simulink model "Zad2manipulator"  (R2025a)
settings: Solver=VariableStepAuto  StartTime=0.0  StopTime=10  RelTol=1e-3
values from neighbouring files (symbols this model uses):
  B1 = 2    [Zad2_manipulator.m]
  B2 = 2    [Zad2_manipulator.m]
  final_uhol = -pi/4    (= -0.785398163397)    [Zad2_manipulator.m]
  g = 9.81    [Zad2_manipulator.m]
  l1 = 0.25    [Zad2_manipulator.m]
  l2 = 0.25    [Zad2_manipulator.m]
  m1 = 3    [Zad2_manipulator.m]
  m2 = 3    [Zad2_manipulator.m]
libraries: slpidlib x2
settings Model: Creator=MATÚŠ  LastModifiedBy=MATÚŠ

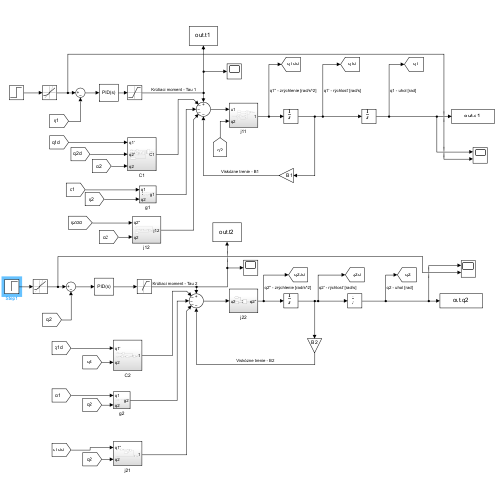
[thumbnail: Simulink's stored preview of the top-level diagram]
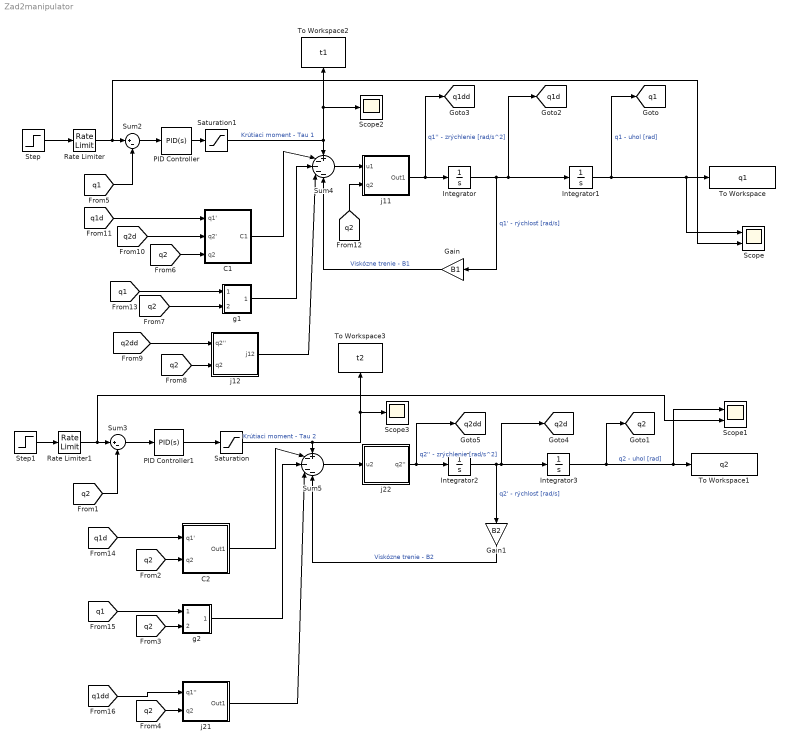
== system Zad2manipulator ==
  C1 : Subsystem
  C2 : Subsystem
  Gain : Gain  Gain=B1
  Gain1 : Gain  Gain=B2
  Integrator : Integrator
  Integrator1 : Integrator  InitialCondition=-pi/2
  Integrator2 : Integrator
  Integrator3 : Integrator  InitialCondition=-pi/2
  PID Controller : slpidlib/PID Controller  Controller=PID  Form=Parallel  TimeDomain=Continuous-time  UseExternalTs=off  SampleTime=-1  IntegratorMethod=Forward Euler  FilterMethod=Forward Euler  ControllerParametersSource=internal  P=300  I=300  UseKiTs=off  D=30  UseExternalDerivativeSource=off  N=300  UseFilter=on  TunerSelectOption=Transfer Function Based (PID Tuner App)  InitialConditionSource=internal  InitialConditionForIntegrator=0  InitialConditionForFilter=0  DifferentiatorICPrevScaledInput=0  ExternalReset=none  TrackingMode=off  Kt=1  LimitOutput=off  SatLimitsSource=internal  UpperSaturationLimit=inf  LowerSaturationLimit=-inf  LinearizeAsGain=on  AntiWindupMode=none  Kb=1  LimitIntegrator=off  UpperIntegratorSaturationLimit=inf  LowerIntegratorSaturationLimit=-inf  POutMin=[]  POutMax=[]  IOutMin=[]  IOutMax=[]  DOutMin=[]  DOutMax=[]  NOutMin=[]  NOutMax=[]  SumOutMin=[]  SumOutMax=[]  SaturationOutMin=[]  SaturationOutMax=[]  PParamMin=[]  PParamMax=[]  IParamMin=[]  IParamMax=[]  DParamMin=[]  DParamMax=[]  NParamMin=[]  NParamMax=[]  KbParamMin=[]  KbParamMax=[]  KtParamMin=[]  KtParamMax=[]  KbOutMin=[]  KbOutMax=[]  KtOutMin=[]  KtOutMax=[]  IntegratorOutMin=[]  IntegratorOutMax=[]  FilterOutMin=[]  FilterOutMax=[]  SumI1OutMin=[]  SumI1OutMax=[]  SumI2OutMin=[]  SumI2OutMax=[]  SumI3OutMin=[]  SumI3OutMax=[]  SumI4OutMin=[]  SumI4OutMax=[]  SumDOutMin=[]  SumDOutMax=[]  DifferentiatorOutMin=[]  DifferentiatorOutMax=[]  FilterDiffOutCoefMin=[]  FilterDiffOutCoefMax=[]  ReciprocalOutMin=[]  ReciprocalOutMax=[]  SumDenOutMin=[]  SumDenOutMax=[]  SumNumOutMin=[]  SumNumOutMax=[]  DivideOutMin=[]  DivideOutMax=[]  UdiffTsProdOutMin=[]  UdiffTsProdOutMax=[]  NTsProdOutMin=[]  NTsProdOutMax=[]  UintegralTsProdOutMin=[]  UintegralTsProdOutMax=[]  UngainTsProdOutMin=[]  UngainTsProdOutMax=[]  ClampingZeroOutDataTypeStr=Inherit: Inherit via back propagation  ClampingZeroOutMin=[]  ClampingZeroOutMax=[]  FilterDenConstantOutDataTypeStr=Inherit: Inherit via back propagation  FilterDenConstantOutMin=[]  FilterDenConstantOutMax=[]  PCopyOutDataTypeStr=Inherit: Inherit via back propagation  PCopyOutMin=[]  PCopyOutMax=[]  NCopyOutDataTypeStr=Inherit: Inherit via back propagation  NCopyOutMin=[]  NCopyOutMax=[]  IntegratorContinuousStateAttributes=''  IntegratorStateMustResolveToSignalObject=off  IntegratorRTWStateStorageClass=Auto  FilterContinuousStateAttributes=''  FilterStateMustResolveToSignalObject=off  FilterRTWStateStorageClass=Auto  ParallelPVariant=InternalParameters  IdealPVariant=Disabled  IVariant=InternalParameters  DVariant=InternalParameters  IntegratorVariant=Continuous  SatVariant=Disabled  AWVariant=Passthrough  PCopyVariant=Disabled  TRVariant=Disabled  FdbkBlocksVariant=Forward  IdealPFdbkVariant=Disabled  SatFdbkVariant=Disabled  DerivativeFilterVariant=ContFilter  NVariant=InternalParameters  NCopyVariant=Disabled  FilterICVariant=InternalICsFilter  IntegratorICVariant=InternalICs  ExternalResetVariant=Disabled  TRSumVariant=Passthrough  SumFdbkVariant=Disabled  SumVariant=Sum_PID  TsampFilterVariant=InternalTs  TsampNgainVariant=Passthrough  TsampIntegralVariant=Disabled_SignalSpec  ExternalSaturationOutDataTypeStr=Inherit: Same as second input  DerivativeSourceVariant=ErrorSignal  PreIntVariant=InternalPreInt
  PID Controller1 : slpidlib/PID Controller  Controller=PID  Form=Parallel  TimeDomain=Continuous-time  UseExternalTs=off  SampleTime=-1  IntegratorMethod=Forward Euler  FilterMethod=Forward Euler  ControllerParametersSource=internal  P=300  I=300  UseKiTs=off  D=30  UseExternalDerivativeSource=off  N=300  UseFilter=on  TunerSelectOption=Transfer Function Based (PID Tuner App)  InitialConditionSource=internal  InitialConditionForIntegrator=0  InitialConditionForFilter=0  DifferentiatorICPrevScaledInput=0  ExternalReset=none  TrackingMode=off  Kt=1  LimitOutput=off  SatLimitsSource=internal  UpperSaturationLimit=inf  LowerSaturationLimit=-inf  LinearizeAsGain=on  AntiWindupMode=none  Kb=1  LimitIntegrator=off  UpperIntegratorSaturationLimit=inf  LowerIntegratorSaturationLimit=-inf  POutMin=[]  POutMax=[]  IOutMin=[]  IOutMax=[]  DOutMin=[]  DOutMax=[]  NOutMin=[]  NOutMax=[]  SumOutMin=[]  SumOutMax=[]  SaturationOutMin=[]  SaturationOutMax=[]  PParamMin=[]  PParamMax=[]  IParamMin=[]  IParamMax=[]  DParamMin=[]  DParamMax=[]  NParamMin=[]  NParamMax=[]  KbParamMin=[]  KbParamMax=[]  KtParamMin=[]  KtParamMax=[]  KbOutMin=[]  KbOutMax=[]  KtOutMin=[]  KtOutMax=[]  IntegratorOutMin=[]  IntegratorOutMax=[]  FilterOutMin=[]  FilterOutMax=[]  SumI1OutMin=[]  SumI1OutMax=[]  SumI2OutMin=[]  SumI2OutMax=[]  SumI3OutMin=[]  SumI3OutMax=[]  SumI4OutMin=[]  SumI4OutMax=[]  SumDOutMin=[]  SumDOutMax=[]  DifferentiatorOutMin=[]  DifferentiatorOutMax=[]  FilterDiffOutCoefMin=[]  FilterDiffOutCoefMax=[]  ReciprocalOutMin=[]  ReciprocalOutMax=[]  SumDenOutMin=[]  SumDenOutMax=[]  SumNumOutMin=[]  SumNumOutMax=[]  DivideOutMin=[]  DivideOutMax=[]  UdiffTsProdOutMin=[]  UdiffTsProdOutMax=[]  NTsProdOutMin=[]  NTsProdOutMax=[]  UintegralTsProdOutMin=[]  UintegralTsProdOutMax=[]  UngainTsProdOutMin=[]  UngainTsProdOutMax=[]  ClampingZeroOutDataTypeStr=Inherit: Inherit via back propagation  ClampingZeroOutMin=[]  ClampingZeroOutMax=[]  FilterDenConstantOutDataTypeStr=Inherit: Inherit via back propagation  FilterDenConstantOutMin=[]  FilterDenConstantOutMax=[]  PCopyOutDataTypeStr=Inherit: Inherit via back propagation  PCopyOutMin=[]  PCopyOutMax=[]  NCopyOutDataTypeStr=Inherit: Inherit via back propagation  NCopyOutMin=[]  NCopyOutMax=[]  IntegratorContinuousStateAttributes=''  IntegratorStateMustResolveToSignalObject=off  IntegratorRTWStateStorageClass=Auto  FilterContinuousStateAttributes=''  FilterStateMustResolveToSignalObject=off  FilterRTWStateStorageClass=Auto  ParallelPVariant=InternalParameters  IdealPVariant=Disabled  IVariant=InternalParameters  DVariant=InternalParameters  IntegratorVariant=Continuous  SatVariant=Disabled  AWVariant=Passthrough  PCopyVariant=Disabled  TRVariant=Disabled  FdbkBlocksVariant=Forward  IdealPFdbkVariant=Disabled  SatFdbkVariant=Disabled  DerivativeFilterVariant=ContFilter  NVariant=InternalParameters  NCopyVariant=Disabled  FilterICVariant=InternalICsFilter  IntegratorICVariant=InternalICs  ExternalResetVariant=Disabled  TRSumVariant=Passthrough  SumFdbkVariant=Disabled  SumVariant=Sum_PID  TsampFilterVariant=InternalTs  TsampNgainVariant=Passthrough  TsampIntegralVariant=Disabled_SignalSpec  ExternalSaturationOutDataTypeStr=Inherit: Same as second input  DerivativeSourceVariant=ErrorSignal  PreIntVariant=InternalPreInt
  Rate Limiter : RateLimiter  SampleTimeMode=inherited
  Rate Limiter1 : RateLimiter  SampleTimeMode=inherited
  Saturation : Saturate  UpperLimit=15  LowerLimit=-15
  Saturation1 : Saturate  UpperLimit=30  LowerLimit=-30
  Scope : Scope  NumInputPorts=2
      settings: ActiveDisplayYMinimum=-1  ActiveDisplayYMaximum=1
  Scope1 : Scope  NumInputPorts=2
      settings: ActiveDisplayYMinimum=-1.2681933125497675  ActiveDisplayYMaximum=0.63598203377017948
  Scope2 : Scope
      settings: ActiveDisplayYMinimum=-1  ActiveDisplayYMaximum=1  DataLoggingVariableName=ScopeData2
  Scope3 : Scope
      settings: DataLoggingVariableName=ScopeData3
  Step : Step  Time=pi/4  Before=-pi/2  After=final_uhol  SampleTime=0
  Step1 : Step  Time=pi/4  Before=-pi/2  After=final_uhol  SampleTime=0
  Sum2 : Sum  Inputs=|+-
  Sum3 : Sum  Inputs=|+-
  Sum4 : Sum  Inputs=+----
  Sum5 : Sum  Inputs=+----
  To Workspace : ToWorkspace  VariableName=q1  SaveFormat=Structure With Time  SampleTime=-1
  To Workspace1 : ToWorkspace  VariableName=q2  SaveFormat=Structure With Time  SampleTime=-1
  To Workspace2 : ToWorkspace  VariableName=t1  SaveFormat=Structure With Time  SampleTime=-1
  To Workspace3 : ToWorkspace  VariableName=t2  SaveFormat=Structure With Time  SampleTime=-1
  g1 : Subsystem
  g2 : Subsystem
  j11 : Subsystem
  j12 : Subsystem
  j21 : Subsystem
  j22 : Subsystem
  tag scope: q1=global, q1d=global, q1dd=global, q2=global, q2d=global, q2dd=global
  wires:
  Sum4/1 -> j11/1(u1)
  Integrator/1 -> [q1d], Integrator1/1, Gain/1  "q1' - rýchlosť [rad/s]"
  Gain1/1 -> Sum5/5  "Viskózne trenie - B2"
  Sum5/1 -> j22/1(u2)
  j22/1(q2'') -> Integrator2/1, [q2dd]  "q2'' - zrýchlenie [rad/s^2]"
  Integrator2/1 -> Integrator3/1, [q2d], Gain1/1  "q2' - rýchlosť [rad/s]"
  Integrator1/1 -> To Workspace/1, Scope/1, [q1]  "q1 - uhol [rad]"
  Integrator3/1 -> Scope1/1, To Workspace1/1, [q2]  "q2 - uhol [rad]"
  j11/1(Out1) -> [q1dd], Integrator/1  "q1'' - zrýchlenie [rad/s^2]"
  [q2] -> C2/2(q2)
  [q2] -> g2/2(q2)
  [q2] -> j21/2(q2)
  [q2] -> C1/3(q2)
  [q2] -> g1/2(q2)
  [q2] -> j12/2(q2)
  [q2dd] -> j12/1(q2'')
  [q2d] -> C1/2(q2')
  [q1d] -> C1/1(q1')
  [q2] -> j11/2(q2)
  [q1] -> g1/1(q1)
  [q1d] -> C2/1(q1')
  [q1] -> g2/1(q1)
  [q1dd] -> j21/1(q1'')
  Gain/1 -> Sum4/5  "Viskózne trenie - B1"
  PID Controller1/1 -> Saturation/1
  Sum3/1 -> PID Controller1/1
  Rate Limiter1/1 -> Scope1/2, Sum3/1
  Step1/1 -> Rate Limiter1/1
  [q2] -> Sum3/2
  Saturation/1 -> Scope3/1, To Workspace3/1, Sum5/1  "Krútiaci moment - Tau 2"
  Sum2/1 -> PID Controller/1
  Rate Limiter/1 -> Sum2/1, Scope/2
  Step/1 -> Rate Limiter/1
  PID Controller/1 -> Saturation1/1
  [q1] -> Sum2/2
  Saturation1/1 -> Sum4/1, To Workspace2/1, Scope2/1  "Krútiaci moment - Tau 1"
  C1/1(C1) -> Sum4/2
  g1/1(g1) -> Sum4/3
  j12/1(j12) -> Sum4/4
  j21/1(Out1) -> Sum5/4
  g2/1(g2) -> Sum5/3
  C2/1(Out1) -> Sum5/2

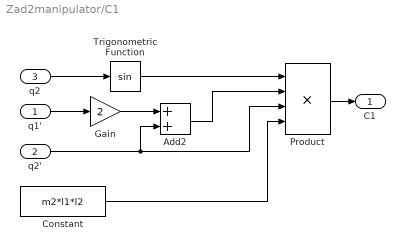
== system Zad2manipulator/C1 ==
  q1' : Inport
  q2' : Inport  Port=2
  q2 : Inport  Port=3
  Add2 : Sum
  Constant : Constant  Value=m2*l1*l2
  Gain : Gain  Gain=2
  Product : Product  Inputs=4
  Trigonometric Function : Trigonometry
  C1 : Outport
  wires:
  Gain/1 -> Add2/1
  Trigonometric Function/1 -> Product/1
  Add2/1 -> Product/2
  Product/1 -> C1/1
  q1'/1 -> Gain/1
  q2'/1 -> Add2/2, Product/3
  q2/1 -> Trigonometric Function/1
  Constant/1 -> Product/4

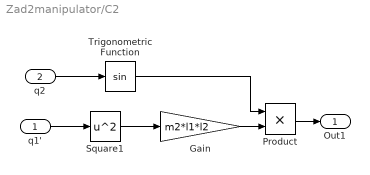
== system Zad2manipulator/C2 ==
  q1' : Inport
  q2 : Inport  Port=2
  Gain : Gain  Gain=m2*l1*l2
  Product : Product
  Square1 : Math  Operator=square
  Trigonometric Function : Trigonometry
  Out1 : Outport
  wires:
  Product/1 -> Out1/1
  Square1/1 -> Gain/1
  Trigonometric Function/1 -> Product/1
  Gain/1 -> Product/2
  q2/1 -> Trigonometric Function/1
  q1'/1 -> Square1/1

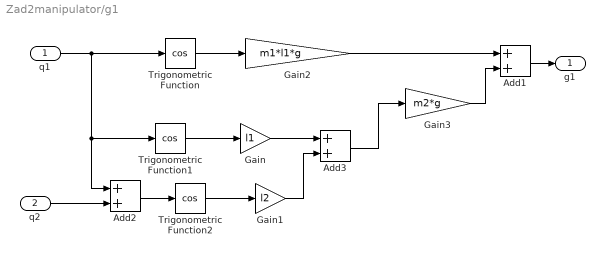
== system Zad2manipulator/g1 ==
  q1 : Inport
  q2 : Inport  Port=2
  Add1 : Sum
  Add2 : Sum
  Add3 : Sum
  Gain : Gain  Gain=l1
  Gain1 : Gain  Gain=l2
  Gain2 : Gain  Gain=m1*l1*g
  Gain3 : Gain  Gain=m2*g
  Trigonometric Function : Trigonometry  Operator=cos
  Trigonometric Function1 : Trigonometry  Operator=cos
  Trigonometric Function2 : Trigonometry  Operator=cos
  g1 : Outport
  wires:
  Add2/1 -> Trigonometric Function2/1
  Add1/1 -> g1/1
  Trigonometric Function1/1 -> Gain/1
  Trigonometric Function2/1 -> Gain1/1
  Gain/1 -> Add3/1
  Gain1/1 -> Add3/2
  Trigonometric Function/1 -> Gain2/1
  Gain2/1 -> Add1/1
  q1/1 -> Trigonometric Function1/1, Add2/1, Trigonometric Function/1
  q2/1 -> Add2/2
  Gain3/1 -> Add1/2
  Add3/1 -> Gain3/1

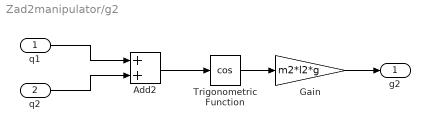
== system Zad2manipulator/g2 ==
  q1 : Inport
  q2 : Inport  Port=2
  Add2 : Sum
  Gain : Gain  Gain=m2*l2*g
  Trigonometric Function : Trigonometry  Operator=cos
  g2 : Outport
  wires:
  Add2/1 -> Trigonometric Function/1
  Gain/1 -> g2/1
  Trigonometric Function/1 -> Gain/1
  q2/1 -> Add2/2
  q1/1 -> Add2/1

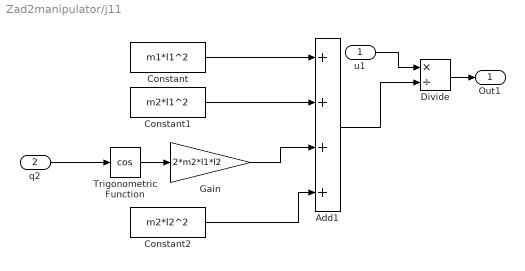
== system Zad2manipulator/j11 ==
  u1 : Inport
  q2 : Inport  Port=2
  Add1 : Sum  Inputs=++++
  Constant : Constant  Value=m1*l1^2
  Constant1 : Constant  Value=m2*l1^2
  Constant2 : Constant  Value=m2*l2^2
  Divide : Product  Inputs=*/
  Gain : Gain  Gain=2*m2*l1*l2
  Trigonometric Function : Trigonometry  Operator=cos
  Out1 : Outport
  wires:
  Add1/1 -> Divide/2
  u1/1 -> Divide/1
  Divide/1 -> Out1/1
  Constant/1 -> Add1/1
  Constant1/1 -> Add1/2
  Trigonometric Function/1 -> Gain/1
  q2/1 -> Trigonometric Function/1
  Gain/1 -> Add1/3
  Constant2/1 -> Add1/4

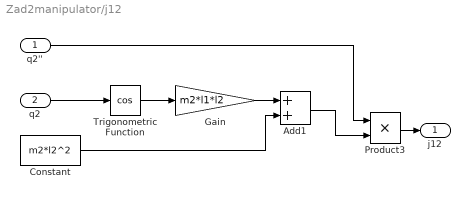
== system Zad2manipulator/j12 ==
  q2'' : Inport
  q2 : Inport  Port=2
  Add1 : Sum
  Constant : Constant  Value=m2*l2^2
  Gain : Gain  Gain=m2*l1*l2
  Product3 : Product
  Trigonometric Function : Trigonometry  Operator=cos
  j12 : Outport
  wires:
  q2/1 -> Trigonometric Function/1
  Trigonometric Function/1 -> Gain/1
  Product3/1 -> j12/1
  Gain/1 -> Add1/1
  Constant/1 -> Add1/2
  Add1/1 -> Product3/2
  q2''/1 -> Product3/1

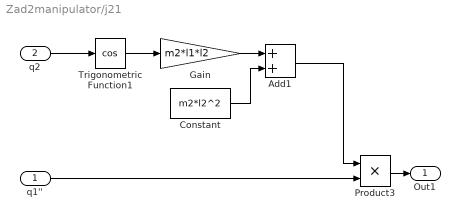
== system Zad2manipulator/j21 ==
  q1'' : Inport
  q2 : Inport  Port=2
  Add1 : Sum
  Constant : Constant  Value=m2*l2^2
  Gain : Gain  Gain=m2*l1*l2
  Product3 : Product
  Trigonometric Function1 : Trigonometry  Operator=cos
  Out1 : Outport
  wires:
  Add1/1 -> Product3/1
  q1''/1 -> Product3/2
  Product3/1 -> Out1/1
  Trigonometric Function1/1 -> Gain/1
  Constant/1 -> Add1/2
  Gain/1 -> Add1/1
  q2/1 -> Trigonometric Function1/1

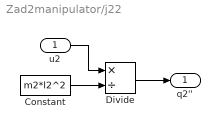
== system Zad2manipulator/j22 ==
  u2 : Inport
  Constant : Constant  Value=m2*l2^2
  Divide : Product  Inputs=*/
  q2'' : Outport
  wires:
  u2/1 -> Divide/1
  Divide/1 -> q2''/1
  Constant/1 -> Divide/2
